simulink model "saw2square"  (R2021b)
settings: Solver=VariableStepAuto  StartTime=0.0  StopTime=10.0  RelTol=1e-3
settings Model: Creator=86195  LastModifiedBy=86195

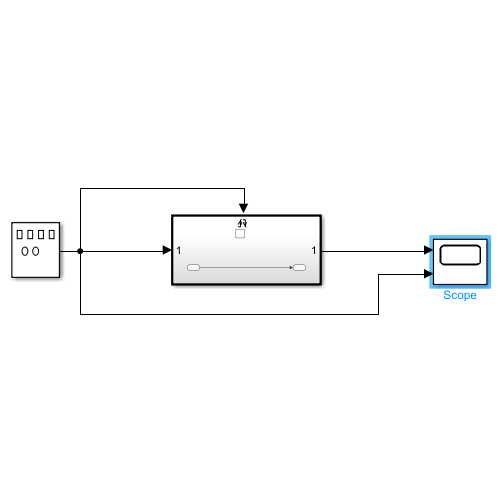
[thumbnail: Simulink's stored preview of the top-level diagram]
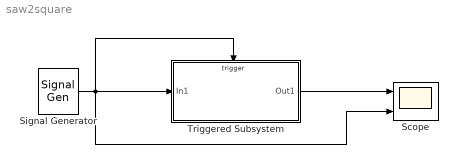
== system saw2square ==
  Scope : Scope  NumInputPorts=2
  Signal Generator : SignalGenerator  WaveForm=sawtooth  Amplitude=4
  Triggered Subsystem : Subsystem  TreatAsAtomicUnit=on
  wires:
  Signal Generator/1 -> Triggered Subsystem/Trigger, Scope/2, Triggered Subsystem/1(In1)
  Triggered Subsystem/1(Out1) -> Scope/1

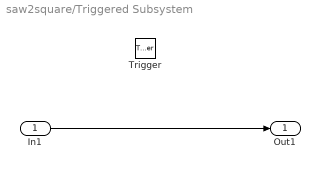
== system saw2square/Triggered Subsystem ==
  In1 : Inport
  Trigger : TriggerPort  TriggerType=either  VariantControl=(inherit)
  Out1 : Outport
  wires:
  In1/1 -> Out1/1
